simulink model "flightgear_dem"  (Simulink 7.8)
settings: Solver=ode45  StartTime=0.0  StopTime=10.0  RelTol=1e-3
libraries: aerolibfltsims x2, aerolibanimutils x1
settings Model: Creator=Dan  LastModifiedBy=Dan

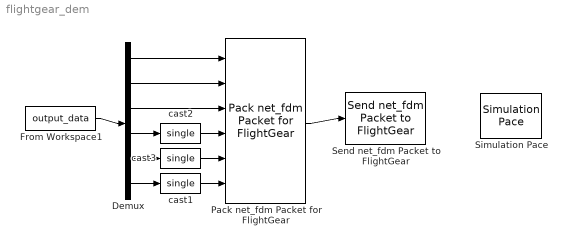
== system flightgear_dem ==
  Demux : Demux  Outputs=6
  From Workspace1 : FromWorkspace  VariableName=output_data  SampleTime=0
  Pack net_fdm Packet for FlightGear : aerolibfltsims/Pack net_fdm Packet for FlightGear  FlightGearVersion=v2.0  ShowPositionAttitudeInputs=on  ShowVelocityAccelerationInputs=off  ShowControlSurfacePositionInputs=off  ShowEngineFuelInputs=off  ShowLandingGearInputs=off  ShowEnvironmentInputs=off  SampleTime=1/30
  Send net_fdm Packet to FlightGear : aerolibfltsims/Send net_fdm Packet to FlightGear  DestinationIpAddress=127.0.0.1  DestinationPort=5502  LocalIpPort=-1  varLen=off  SampleTime=1/30
  Simulation Pace : aerolibanimutils/Simulation Pace  SimulationPace=1  SleepMode=MATLAB Thread  OutputPaceError=off  SampleTime=0.001
      settings: AttributesFormatString=%<SimulationPace> sec/sec
  cast1 : DataTypeConversion  OutDataTypeStr=single  SaturateOnIntegerOverflow=on
  cast2 : DataTypeConversion  OutDataTypeStr=single  SaturateOnIntegerOverflow=on
  cast3 : DataTypeConversion  OutDataTypeStr=single  SaturateOnIntegerOverflow=on
  wires:
  Pack net_fdm Packet for FlightGear/1 -> Send net_fdm Packet to FlightGear/1
  Demux/1 -> Pack net_fdm Packet for FlightGear/1
  From Workspace1/1 -> Demux/1
  Demux/4 -> cast2/1
  Demux/5 -> cast3/1
  Demux/6 -> cast1/1
  Demux/2 -> Pack net_fdm Packet for FlightGear/2
  Demux/3 -> Pack net_fdm Packet for FlightGear/3
  cast2/1 -> Pack net_fdm Packet for FlightGear/4
  cast3/1 -> Pack net_fdm Packet for FlightGear/5
  cast1/1 -> Pack net_fdm Packet for FlightGear/6
